simulink model "ROVModelp"  (R2017a)
settings: Solver=VariableStepAuto  StartTime=0.0  StopTime=250  RelTol=1e-3
settings Model: Creator=varunpwr  LastModifiedBy=varunpwr

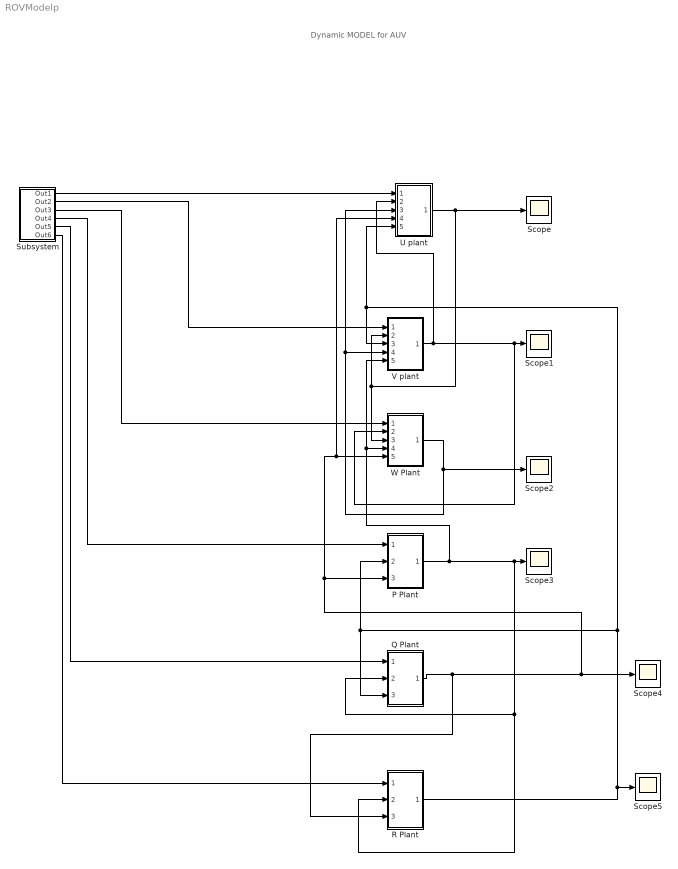
== system ROVModelp ==
  note: Dynamic MODEL for AUV
  P Plant : Subsystem
  Q Plant : Subsystem
  "R Plant " : Subsystem
  Scope{,1..5} (6 alike) : Scope
  Subsystem : Subsystem
  "U plant " : Subsystem
  "V plant " : Subsystem
  "W Plant " : Subsystem
  wires:
  Subsystem/1(Out1) -> "U plant "/1(In1)
  "U plant "/1(Out1) -> "V plant "/2(In2), "W Plant "/3(In3), Scope/1
  Subsystem/2(Out2) -> "V plant "/1(In1)
  "V plant "/1(Out1) -> "W Plant "/2(In2), Scope1/1, "U plant "/2(In2)
  "W Plant "/1(Out1) -> Scope2/1, "V plant "/4(In4), "U plant "/3(In3)
  Subsystem/3(Out3) -> "W Plant "/1(In1)
  P Plant/1(Out1) -> "R Plant "/2(In2), Q Plant/2(In2), Scope3/1, "W Plant "/4(In4), "V plant "/5(In5)
  Subsystem/4(Out4) -> P Plant/1(In1)
  Q Plant/1(Out1) -> Scope4/1, P Plant/3("In3 "), "W Plant "/5(In5), "U plant "/4(In4), "R Plant "/3(In3)
  Subsystem/5(Out5) -> Q Plant/1(In1)
  "R Plant "/1(Out1) -> Scope5/1, Q Plant/3(In3), P Plant/2(In2), "V plant "/3(In3), "U plant "/5(In5)
  Subsystem/6(Out6) -> "R Plant "/1(In1)

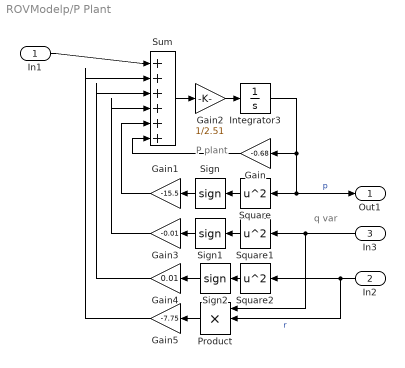
== system ROVModelp/P Plant ==
  note: q var
  note: P plant
  In1 : Inport
  In2 : Inport  Port=2
  "In3 " : Inport  Port=3
  Gain : Gain  Gain=-0.68
  Gain1 : Gain  Gain=-15.5
  Gain2 : Gain  Gain=1/2.51
  Gain3 : Gain  Gain=-0.01
  Gain4 : Gain  Gain=0.01
  Gain5 : Gain  Gain=-7.75
  Integrator3 : Integrator
  Product : Product  Inputs=3
  Sign : Signum
  Sign1 : Signum
  Sign2 : Signum
  Square : Math  Operator=square  SaturateOnIntegerOverflow=on
  Square1 : Math  Operator=square  SaturateOnIntegerOverflow=on
  Square2 : Math  Operator=square  SaturateOnIntegerOverflow=on
  Sum : Sum  Inputs=++++|++
  Out1 : Outport
  wires:
  Product/1 -> Gain5/1
  Sum/1 -> Gain2/1
  Gain3/1 -> Sum/4
  Gain4/1 -> Sum/3
  Gain2/1 -> Integrator3/1
  In1/1 -> Sum/1
  Gain5/1 -> Sum/2
  "In3 "/1 -> Product/1, Square1/1
  Gain1/1 -> Sum/5
  Gain/1 -> Sum/6
  In2/1 -> Product/2, Square2/1  "r"
  Integrator3/1 -> Out1/1, Square/1, Gain/1  "p"
  Sign/1 -> Gain1/1
  Square/1 -> Sign/1
  Sign1/1 -> Gain3/1
  Square1/1 -> Sign1/1
  Sign2/1 -> Gain4/1
  Square2/1 -> Sign2/1

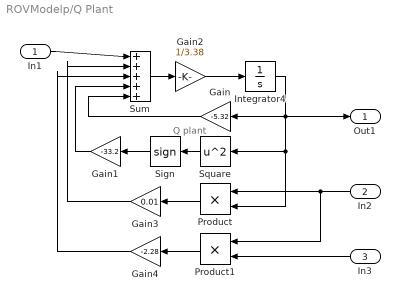
== system ROVModelp/Q Plant ==
  note: Q plant
  In1 : Inport
  In2 : Inport  Port=2
  In3 : Inport  Port=3
  Gain : Gain  Gain=-5.32
  Gain1 : Gain  Gain=-33.2
  Gain2 : Gain  Gain=1/3.38
  Gain3 : Gain  Gain=0.01
  Gain4 : Gain  Gain=-2.28
  Integrator4 : Integrator
  Product : Product
  Product1 : Product
  Sign : Signum
  Square : Math  Operator=square  SaturateOnIntegerOverflow=on
  Sum : Sum  Inputs=+++|++
  Out1 : Outport
  wires:
  Gain1/1 -> Sum/4
  In2/1 -> Product/1, Product1/1
  Gain4/1 -> Sum/3
  In3/1 -> Product1/2
  In1/1 -> Sum/1
  Product/1 -> Gain3/1
  Integrator4/1 -> Out1/1, Square/1, Product/2, Gain/1
  Gain/1 -> Sum/5
  Gain2/1 -> Integrator4/1
  Sum/1 -> Gain2/1
  Product1/1 -> Gain4/1
  Gain3/1 -> Sum/2
  Sign/1 -> Gain1/1
  Square/1 -> Sign/1

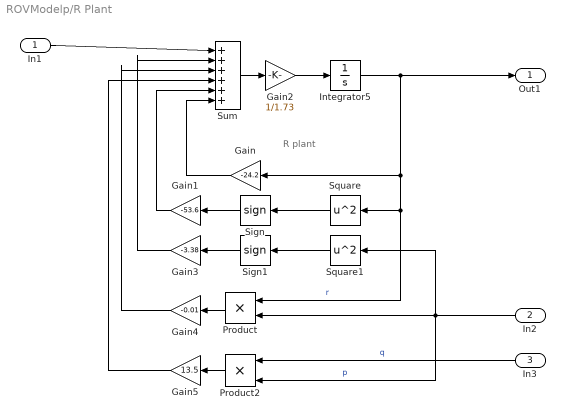
== system ROVModelp/R Plant  ==
  note: R plant
  In1 : Inport
  In2 : Inport  Port=2
  In3 : Inport  Port=3
  Gain : Gain  Gain=-24.2
  Gain1 : Gain  Gain=-53.6
  Gain2 : Gain  Gain=1/1.73
  Gain3 : Gain  Gain=-3.38
  Gain4 : Gain  Gain=-0.01
  Gain5 : Gain  Gain=13.5
  Integrator5 : Integrator
  Product : Product
  Product2 : Product  Inputs=3
  Sign : Signum
  Sign1 : Signum
  Square : Math  Operator=square  SaturateOnIntegerOverflow=on
  Square1 : Math  Operator=square  SaturateOnIntegerOverflow=on
  Sum : Sum  Inputs=+++|+++
  Out1 : Outport
  wires:
  Product/1 -> Gain4/1
  Gain3/1 -> Sum/2
  Gain4/1 -> Sum/3
  Integrator5/1 -> Product/1, Square/1, Gain/1, Out1/1  "r"
  In2/1 -> Product2/3, Square1/1, Product/2  "p"
  Gain1/1 -> Sum/5
  In3/1 -> Product2/1  "q"
  Gain/1 -> Sum/6
  Gain2/1 -> Integrator5/1
  Product2/1 -> Gain5/1
  Sum/1 -> Gain2/1
  In1/1 -> Sum/1
  Gain5/1 -> Sum/4
  Sign/1 -> Gain1/1
  Square/1 -> Sign/1
  Sign1/1 -> Gain3/1
  Square1/1 -> Sign1/1

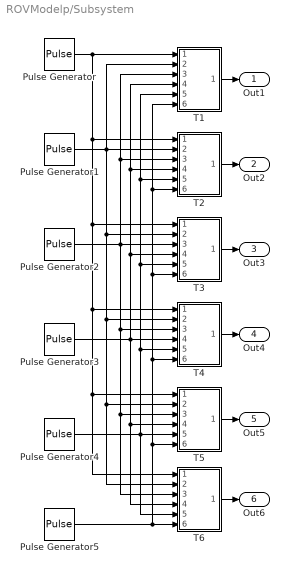
== system ROVModelp/Subsystem ==
  Pulse Generator : DiscretePulseGenerator  PulseType=Time based  Period=10  PulseWidth=5
  Pulse Generator{1..2,4..5} (4 alike) : DiscretePulseGenerator  PulseType=Time based  Amplitude=0  Period=10  PulseWidth=5
  Pulse Generator3 : DiscretePulseGenerator  PulseType=Time based  Amplitude=100  Period=50  PulseWidth=5
  "T1 " : Subsystem
  T2 : Subsystem
  "T3 " : Subsystem
  T4 : Subsystem
  T5 : Subsystem
  T6 : Subsystem
  Out1 : Outport
  Out2 : Outport  Port=2
  Out3 : Outport  Port=3
  Out4 : Outport  Port=4
  Out5 : Outport  Port=5
  Out6 : Outport  Port=6
  wires:
  "T3 "/1(Out1) -> Out3/1
  "T1 "/1(Out1) -> Out1/1
  T6/1(Out1) -> Out6/1
  T4/1(Out1) -> Out4/1
  Pulse Generator5/1 -> "T1 "/6(In6), T2/6(In6), "T3 "/6(In6), T4/6(In6), T5/6(In6), T6/6(In6)
  T2/1(Out1) -> Out2/1
  T5/1(Out1) -> Out5/1
  Pulse Generator3/1 -> T4/4(In4), T6/4(In4), T5/4(In4), "T3 "/4(In4), T2/4(In4), "T1 "/4(In4)
  Pulse Generator4/1 -> T6/5(In5), T5/5(In5), T4/5(In5), "T3 "/5(In5), T2/5(In5), "T1 "/5(In5)
  Pulse Generator1/1 -> "T3 "/2(In2), T4/2(In2), T5/2(In2), T6/2(In2), T2/2(In2), "T1 "/2(In2)
  Pulse Generator2/1 -> T4/3(In3), T5/3(In3), T6/3(In3), "T3 "/3(In3), "T1 "/3(In3), T2/3(In3)
  Pulse Generator/1 -> T2/1(In1), "T3 "/1(In1), T4/1(In1), T5/1(In1), T6/1(In1), "T1 "/1(In1)

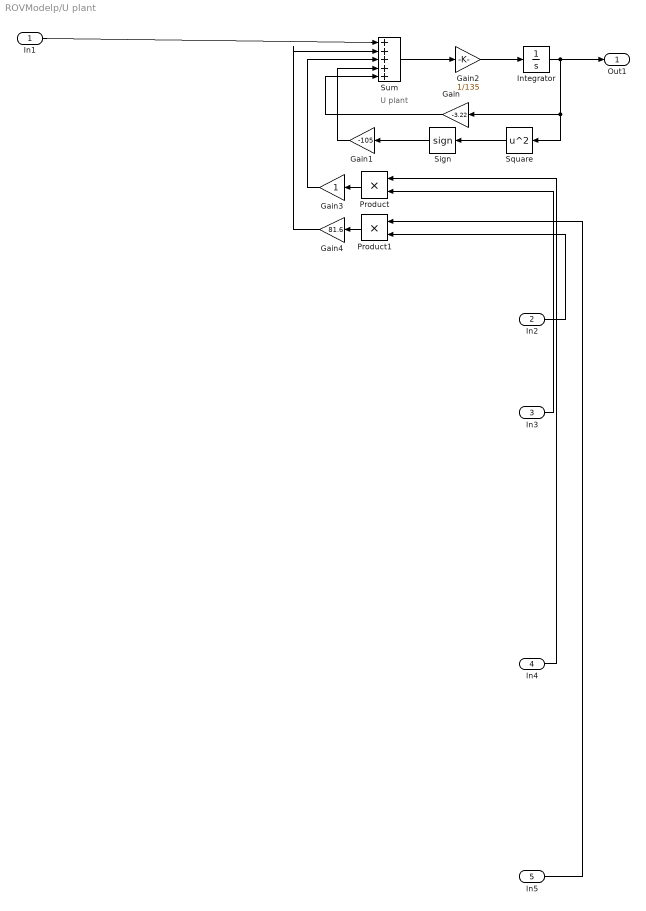
== system ROVModelp/U plant  ==
  note: U plant
  In1 : Inport
  In2 : Inport  Port=2
  In3 : Inport  Port=3
  In4 : Inport  Port=4
  In5 : Inport  Port=5
  Gain : Gain  Gain=-3.22
  Gain1 : Gain  Gain=-105
  Gain2 : Gain  Gain=1/135
  Gain3 : Gain
  Gain4 : Gain  Gain=81.6
  Integrator : Integrator
  Product : Product
  Product1 : Product
  Sign : Signum
  Square : Math  Operator=square  SaturateOnIntegerOverflow=on
  Sum : Sum  Inputs=++|+++
  Out1 : Outport
  wires:
  Gain4/1 -> Sum/2
  In2/1 -> Product1/2
  Sum/1 -> Gain2/1
  In4/1 -> Product/1
  Product/1 -> Gain3/1
  Gain3/1 -> Sum/3
  In5/1 -> Product1/1
  In1/1 -> Sum/1
  Integrator/1 -> Out1/1, Square/1, Gain/1
  Gain2/1 -> Integrator/1
  Product1/1 -> Gain4/1
  In3/1 -> Product/2
  Gain/1 -> Sum/5
  Gain1/1 -> Sum/4
  Square/1 -> Sign/1
  Sign/1 -> Gain1/1

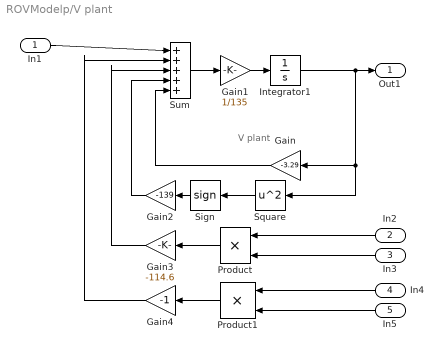
== system ROVModelp/V plant  ==
  note: V plant
  In1 : Inport
  In2 : Inport  Port=2
  In3 : Inport  Port=3
  In4 : Inport  Port=4
  In5 : Inport  Port=5
  Gain : Gain  Gain=-3.29
  Gain1 : Gain  Gain=1/135
  Gain2 : Gain  Gain=-139
  Gain3 : Gain  Gain=-114.6
  Gain4 : Gain  Gain=-1
  Integrator1 : Integrator
  Product : Product
  Product1 : Product
  Sign : Signum
  Square : Math  Operator=square  SaturateOnIntegerOverflow=on
  Sum : Sum  Inputs=+++|++
  Out1 : Outport
  wires:
  Gain2/1 -> Sum/4
  Product/1 -> Gain3/1
  In5/1 -> Product1/2
  In2/1 -> Product/1
  In3/1 -> Product/2
  Integrator1/1 -> Square/1, Gain/1, Out1/1
  In4/1 -> Product1/1
  Gain3/1 -> Sum/3
  Sum/1 -> Gain1/1
  Gain/1 -> Sum/5
  Gain1/1 -> Integrator1/1
  In1/1 -> Sum/1
  Gain4/1 -> Sum/2
  Product1/1 -> Gain4/1
  Square/1 -> Sign/1
  Sign/1 -> Gain2/1

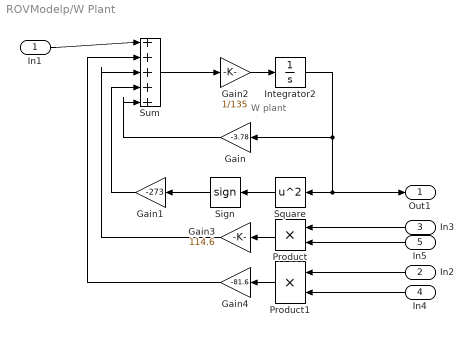
== system ROVModelp/W Plant  ==
  note: W plant
  In1 : Inport
  In2 : Inport  Port=2
  In3 : Inport  Port=3
  In4 : Inport  Port=4
  In5 : Inport  Port=5
  Gain : Gain  Gain=-3.78
  Gain1 : Gain  Gain=-273
  Gain2 : Gain  Gain=1/135
  Gain3 : Gain  Gain=114.6
  Gain4 : Gain  Gain=-81.6
  Integrator2 : Integrator
  Product : Product
  Product1 : Product
  Sign : Signum
  Square : Math  Operator=square  SaturateOnIntegerOverflow=on
  Sum : Sum  Inputs=+++|++
  Out1 : Outport
  wires:
  Gain3/1 -> Sum/3
  Gain/1 -> Sum/5
  Gain1/1 -> Sum/4
  In1/1 -> Sum/1
  Gain2/1 -> Integrator2/1
  Product/1 -> Gain3/1
  In2/1 -> Product1/1
  Integrator2/1 -> Out1/1, Square/1, Gain/1
  Sum/1 -> Gain2/1
  In3/1 -> Product/1
  Product1/1 -> Gain4/1
  Gain4/1 -> Sum/2
  In4/1 -> Product1/2
  In5/1 -> Product/2
  Square/1 -> Sign/1
  Sign/1 -> Gain1/1

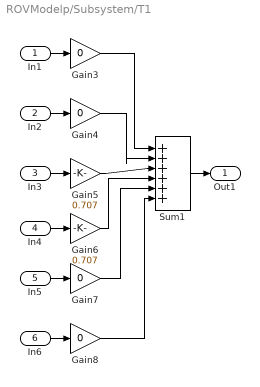
== system ROVModelp/Subsystem/T1  ==
  In1 : Inport
  In2 : Inport  Port=2
  In3 : Inport  Port=3
  In4 : Inport  Port=4
  In5 : Inport  Port=5
  In6 : Inport  Port=6
  Gain{3..4,7..8} (4 alike) : Gain  Gain=0
  Gain5 : Gain  Gain=0.707
  Gain6 : Gain  Gain=0.707
  Sum1 : Sum  Inputs=+|+++++
  Out1 : Outport
  wires:
  Gain6/1 -> Sum1/4
  Sum1/1 -> Out1/1
  Gain4/1 -> Sum1/2
  In6/1 -> Gain8/1
  In3/1 -> Gain5/1
  In2/1 -> Gain4/1
  Gain5/1 -> Sum1/3
  In1/1 -> Gain3/1
  Gain3/1 -> Sum1/1
  In5/1 -> Gain7/1
  Gain7/1 -> Sum1/5
  Gain8/1 -> Sum1/6
  In4/1 -> Gain6/1

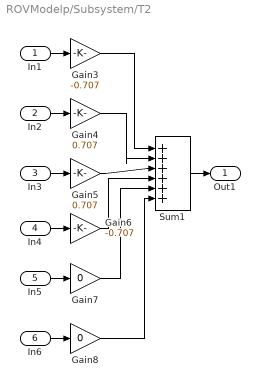
== system ROVModelp/Subsystem/T2 ==
  In1 : Inport
  In2 : Inport  Port=2
  In3 : Inport  Port=3
  In4 : Inport  Port=4
  In5 : Inport  Port=5
  In6 : Inport  Port=6
  Gain3 : Gain  Gain=-0.707
  Gain4 : Gain  Gain=0.707
  Gain5 : Gain  Gain=0.707
  Gain6 : Gain  Gain=-0.707
  Gain7 : Gain  Gain=0
  Gain8 : Gain  Gain=0
  Sum1 : Sum  Inputs=+|+++++
  Out1 : Outport
  wires:
  In4/1 -> Gain6/1
  Gain8/1 -> Sum1/6
  Gain7/1 -> Sum1/5
  In5/1 -> Gain7/1
  Gain3/1 -> Sum1/1
  In1/1 -> Gain3/1
  Gain5/1 -> Sum1/3
  In2/1 -> Gain4/1
  In3/1 -> Gain5/1
  In6/1 -> Gain8/1
  Gain4/1 -> Sum1/2
  Sum1/1 -> Out1/1
  Gain6/1 -> Sum1/4

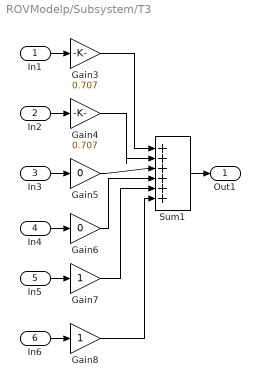
== system ROVModelp/Subsystem/T3  ==
  In1 : Inport
  In2 : Inport  Port=2
  In3 : Inport  Port=3
  In4 : Inport  Port=4
  In5 : Inport  Port=5
  In6 : Inport  Port=6
  Gain3 : Gain  Gain=0.707
  Gain4 : Gain  Gain=0.707
  Gain5 : Gain  Gain=0
  Gain6 : Gain  Gain=0
  Gain7 : Gain
  Gain8 : Gain
  Sum1 : Sum  Inputs=+|+++++
  Out1 : Outport
  wires:
  Gain6/1 -> Sum1/4
  Sum1/1 -> Out1/1
  Gain4/1 -> Sum1/2
  In6/1 -> Gain8/1
  In3/1 -> Gain5/1
  In2/1 -> Gain4/1
  Gain5/1 -> Sum1/3
  In1/1 -> Gain3/1
  Gain3/1 -> Sum1/1
  In5/1 -> Gain7/1
  Gain7/1 -> Sum1/5
  Gain8/1 -> Sum1/6
  In4/1 -> Gain6/1

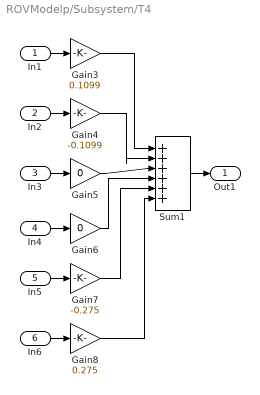
== system ROVModelp/Subsystem/T4 ==
  In1 : Inport
  In2 : Inport  Port=2
  In3 : Inport  Port=3
  In4 : Inport  Port=4
  In5 : Inport  Port=5
  In6 : Inport  Port=6
  Gain3 : Gain  Gain=0.1099
  Gain4 : Gain  Gain=-0.1099
  Gain5 : Gain  Gain=0
  Gain6 : Gain  Gain=0
  Gain7 : Gain  Gain=-0.275
  Gain8 : Gain  Gain=0.275
  Sum1 : Sum  Inputs=+|+++++
  Out1 : Outport
  wires:
  In4/1 -> Gain6/1
  Gain8/1 -> Sum1/6
  Gain7/1 -> Sum1/5
  In5/1 -> Gain7/1
  Gain3/1 -> Sum1/1
  In1/1 -> Gain3/1
  Gain5/1 -> Sum1/3
  In2/1 -> Gain4/1
  In3/1 -> Gain5/1
  In6/1 -> Gain8/1
  Gain4/1 -> Sum1/2
  Sum1/1 -> Out1/1
  Gain6/1 -> Sum1/4

== system ROVModelp/Subsystem/T5 ==
  In1 : Inport
  In2 : Inport  Port=2
  In3 : Inport  Port=3
  In4 : Inport  Port=4
  In5 : Inport  Port=5
  In6 : Inport  Port=6
  Gain3 : Gain  Gain=0.2789
  Gain4 : Gain  Gain=0.2789
  Gain5 : Gain  Gain=0.3044
  Gain6 : Gain  Gain=0.3044
  Gain7 : Gain  Gain=-0.0355
  Gain8 : Gain  Gain=-0.0355
  Sum1 : Sum  Inputs=+|+++++
  Out1 : Outport
  wires:
  Gain6/1 -> Sum1/4
  Sum1/1 -> Out1/1
  Gain4/1 -> Sum1/2
  In6/1 -> Gain8/1
  In3/1 -> Gain5/1
  In2/1 -> Gain4/1
  Gain5/1 -> Sum1/3
  In1/1 -> Gain3/1
  Gain3/1 -> Sum1/1
  In5/1 -> Gain7/1
  Gain7/1 -> Sum1/5
  Gain8/1 -> Sum1/6
  In4/1 -> Gain6/1

== system ROVModelp/Subsystem/T6 ==
  In1 : Inport
  In2 : Inport  Port=2
  In3 : Inport  Port=3
  In4 : Inport  Port=4
  In5 : Inport  Port=5
  In6 : Inport  Port=6
  Gain3 : Gain  Gain=-0.2789
  Gain4 : Gain  Gain=0.2789
  Gain5 : Gain  Gain=-0.467
  Gain6 : Gain  Gain=0.467
  Gain7 : Gain  Gain=0
  Gain8 : Gain  Gain=0
  Sum1 : Sum  Inputs=+|+++++
  Out1 : Outport
  wires:
  In4/1 -> Gain6/1
  Gain8/1 -> Sum1/6
  Gain7/1 -> Sum1/5
  In5/1 -> Gain7/1
  Gain3/1 -> Sum1/1
  In1/1 -> Gain3/1
  Gain5/1 -> Sum1/3
  In2/1 -> Gain4/1
  In3/1 -> Gain5/1
  In6/1 -> Gain8/1
  Gain4/1 -> Sum1/2
  Sum1/1 -> Out1/1
  Gain6/1 -> Sum1/4
